simulink model "newfullgrid"  (R2024b)
settings: Solver=FixedStepDiscrete  StartTime=0.0  StopTime=24  FixedStep=0.0001  MaxStep=Ts  RelTol=1e-3
values from neighbouring files (symbols this model uses):
  C_boost = 1000e-6    (= 0.001)    [Full_system_design.m]    (also in systemdesigncode.m)
  f = 60    [Full_system_design.m]    (also in systemdesigncode.m)
  L_boost = 10*L_bound    (= 0.0016236346)    [Full_system_design.m]    (also in systemdesigncode.m)
  Lf = ((0.1*U^2)/(2*pi*f*(P/3)))    (= 0.00229819737825)    [Full_system_design.m]    (also in systemdesigncode.m)
  PV_power_max = Vpv_out_max * Ipv_out_max    (= 50729.7)    [Full_system_design.m]    (also in systemdesigncode.m)
  SOC_max = 90    [Full_system_design.m]    (also in batteryEnvLogic.m; gridrl.m = 1; systemdesigncode.m)
  SOC_min = 20    [Full_system_design.m]    (also in batteryEnvLogic.m; gridrl.m = 0.2; systemdesigncode.m)
  Solar_Irradiance = data.Solar_Irradiance    [systemdesigncode.m]
  Temperature = data.Temperature    [systemdesigncode.m]
  Ts = 10e-6    (= 1e-05)    [Full_system_design.m]    (also in systemdesigncode.m)
  V_bus_ref = 800    [Full_system_design.m]    (also in systemdesigncode.m)
undefined symbols (not defined in the file or in its folder): Active_Power_kW, Ion, Lithium
libraries: spsSeriesRLCBranchLib x6, slpidlib x4, spsMosfetLib x2, spsPWMGeneratorDCDCLib x2, rllib x2, spsPower3phInstantaneousLib x2, spsThreePhaseVIMeasurementLib x2, spsBatteryLib x1, spsCurrentMeasurementLib x1, spsDiodeLib x1, spsIGBTLib x1, spsPLL3phLib x1
settings Model: SimulationMode=accelerator  Creator=MohamedAbdallahMosta  LastModifiedBy=mac
settings DataIOCC: TimeSaveName=simTime  OutputSaveName=simOutput
settings DebuggingCC: UnconnectedInputMsg=warning  UnconnectedOutputMsg=warning  UnconnectedLineMsg=warning
settings ModelReferenceCC: EnableRefExpFcnMdlSchedulingChecks=on
settings RTWCC: GPUComputeCapability=3.5  DLArmComputeVersion=19.05

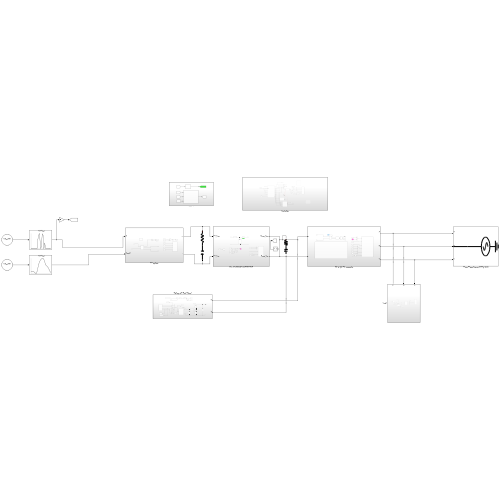
[thumbnail: Simulink's stored preview of the top-level diagram]
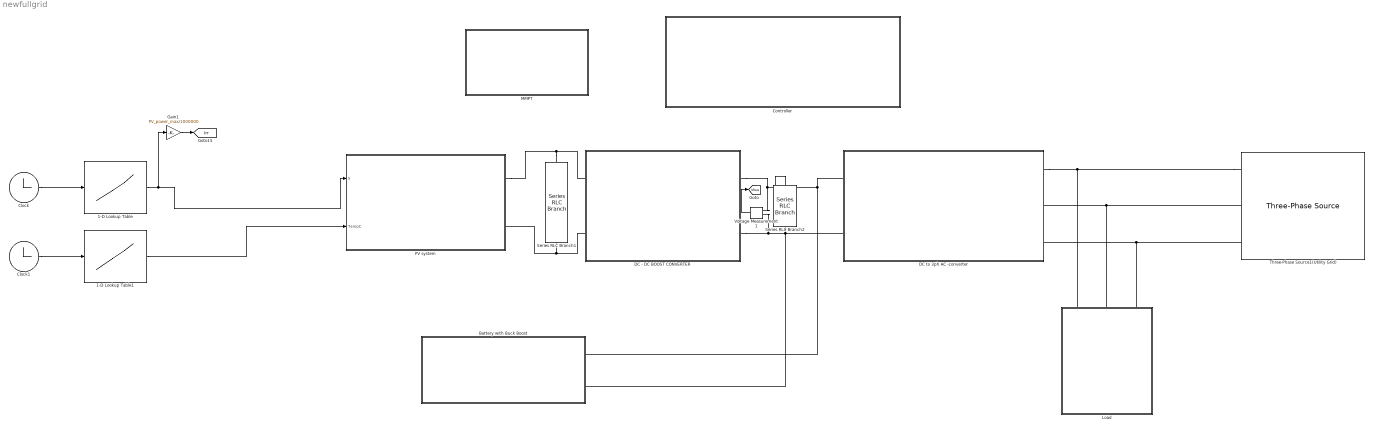
== system newfullgrid ==
  1-D Lookup Table : Lookup_n-D  NumberOfTableDimensions=1  BreakpointsForDimension1=[0:23]  Table=Solar_Irradiance  InternalRulePriority=Speed  RndMeth=Simplest
  1-D Lookup Table1 : Lookup_n-D  NumberOfTableDimensions=1  BreakpointsForDimension1=[0:23]  Table=Temperature  InternalRulePriority=Speed  RndMeth=Simplest
  Battery with Buck Boost : Subsystem
  Clock : Clock
  Clock1 : Clock
  Controller : Subsystem
  DC - DC BOOST CONVERTER : Subsystem
  DC to 3ph AC -converter : Subsystem
  Gain1 : Gain  Gain=PV_power_max/1000000
  Load : Subsystem
  MMPT : Subsystem
  PV system : Subsystem
  Series RLC Branch1 : spsSeriesRLCBranchLib/Series RLC Branch  LConnTagsString=__new0  RConnTagsString=__new0  BranchType=RC  Resistance=1e-4  Inductance=L_boost  SetiL0=off  InitialCurrent=0  Capacitance=100e-6  Setx0=off  InitialVoltage=406  Measurements=None
  Series RLC Branch2 : spsSeriesRLCBranchLib/Series RLC Branch  LConnTagsString=__new0  RConnTagsString=__new0  BranchType=RC  Resistance=1e-4  Inductance=L_boost  SetiL0=off  InitialCurrent=0  Capacitance=C_boost  Setx0=off  InitialVoltage=800  Measurements=None
  Three-Phase Source1(Utility Grid) : spsThreePhaseSourceLib/Three-Phase Source  InternalConnection=Yg  VoltagePhases=off  Voltage=380  PhaseAngle=0  Voltage_phases=[25e3 25e3 25e3]/sqrt(3)  PhaseAngles_phases=[0 -120 +120]  Frequency=f  NonIdealSource=off  SpecifyImpedance=off  Resistance=0.8929  Inductance=16.58e-3  ShortCircuitLevel=100e6  BaseVoltage=25e3  XRratio=7  BusType=swing  Pref=10e3  Qref=0  Prefabc=[10e3, 10e3, 10e3]  Qrefabc=[0, 0, 0]  Qmin=-inf  Qmax=inf
  Voltage Measurement1 : spsVoltageMeasurementLib/Voltage Measurement  PhasorSimulation=off  OutputType=Complex  PSBequivalent=0
  tag scope: Irr=global, Vbus=global
  wires:
  Gain1/1 -> [Irr]
  1-D Lookup Table1/1 -> PV system/2(TempC)
  Clock1/1 -> 1-D Lookup Table1/1
  Clock/1 -> 1-D Lookup Table/1
  1-D Lookup Table/1 -> PV system/1(S), Gain1/1
  Voltage Measurement1/1 -> [Vbus]
  connections:
  DC to 3ph AC -converter/RConn1 -- DC - DC BOOST CONVERTER/RConn1 -- Voltage Measurement1/LConn1 -- Series RLC Branch2/LConn1 -- Battery with Buck Boost/LConn1
  Series RLC Branch2/RConn1 -- Battery with Buck Boost/LConn2 -- DC to 3ph AC -converter/RConn2 -- DC - DC BOOST CONVERTER/RConn2 -- Voltage Measurement1/LConn2
  Series RLC Branch1/LConn1 -- DC - DC BOOST CONVERTER/LConn1 -- PV system/RConn1
  DC to 3ph AC -converter/LConn3 -- Three-Phase Source1(Utility Grid)/RConn3 -- Load/LConn3
  Three-Phase Source1(Utility Grid)/RConn1 -- DC to 3ph AC -converter/LConn1 -- Load/LConn1
  Three-Phase Source1(Utility Grid)/RConn2 -- Load/LConn2 -- DC to 3ph AC -converter/LConn2
  Series RLC Branch1/RConn1 -- DC - DC BOOST CONVERTER/LConn2 -- PV system/RConn2

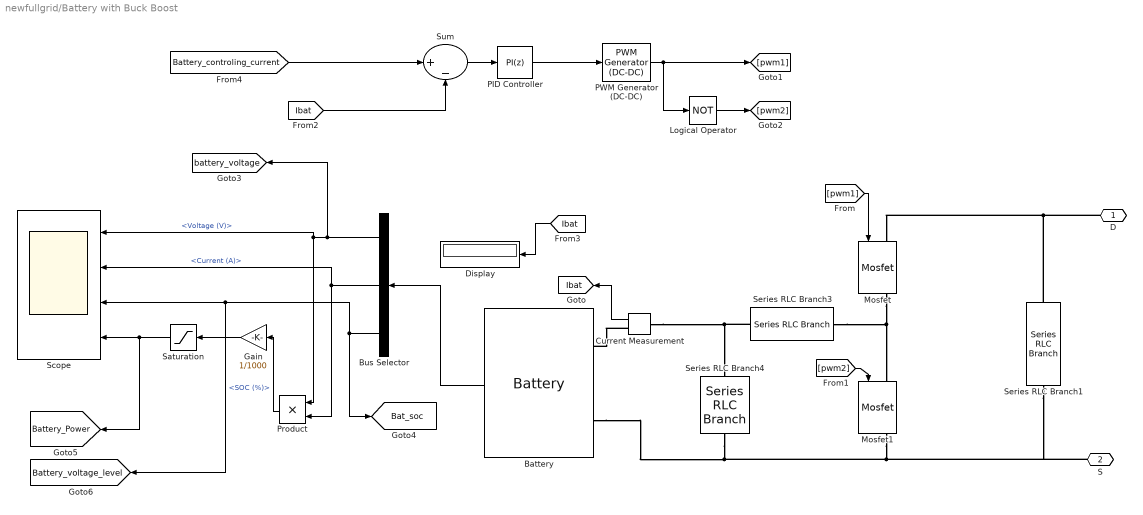
== system newfullgrid/Battery with Buck Boost ==
  Battery : spsBatteryLib/Battery  BatType=Lithium-Ion  NomV=360  NomQ=50  SOC=85  Batt_Tr=1  PresetModel=on  MaxQ=50  MinV=270  FullV=419.0354  Dis_rate=21.7391  R=0.072  Normal_OP=45.2174  expZone="[388.9389      2.456522]"
  Bus Selector : BusSelector  OutputSignals=Voltage (V),Current (A),SOC (%)
  Current Measurement : spsCurrentMeasurementLib/Current Measurement  PhasorSimulation=off  OutputType=Complex  PSBequivalent=0
  Display : Display
  Gain : Gain  Gain=1/1000
  Logical Operator : Logic  Operator=NOT  AllPortsSameDT=off  OutDataTypeStr=boolean
  Mosfet : spsMosfetLib/Mosfet  Ron=0.1  Lon=0  Rd=0.01  Vfd=0  IC=0  Rs=1e5  Cs=inf  Measurements=on
  Mosfet1 : spsMosfetLib/Mosfet  Ron=0.1  Lon=0  Rd=0.01  Vfd=0  IC=0  Rs=1e5  Cs=inf  Measurements=on
  PID Controller : slpidlib/PID Controller  Controller=PI  Form=Parallel  TimeDomain=Discrete-time  UseExternalTs=off  SampleTime=Ts  IntegratorMethod=Forward Euler  FilterMethod=Forward Euler  ControllerParametersSource=internal  P=1.5  I=25  UseKiTs=off  D=0  UseExternalDerivativeSource=off  N=100  UseFilter=on  TunerSelectOption=Transfer Function Based (PID Tuner App)  InitialConditionSource=internal  InitialConditionForIntegrator=0  InitialConditionForFilter=0  DifferentiatorICPrevScaledInput=0  ExternalReset=none  TrackingMode=off  Kt=1  LimitOutput=on  SatLimitsSource=internal  UpperSaturationLimit=0.95  LowerSaturationLimit=0  LinearizeAsGain=on  AntiWindupMode=none  Kb=1  LimitIntegrator=off  UpperIntegratorSaturationLimit=inf  LowerIntegratorSaturationLimit=-inf  POutMin=[]  POutMax=[]  IOutMin=[]  IOutMax=[]  DOutMin=[]  DOutMax=[]  NOutMin=[]  NOutMax=[]  SumOutMin=[]  SumOutMax=[]  SaturationOutMin=[]  SaturationOutMax=[]  PParamMin=[]  PParamMax=[]  IParamMin=[]  IParamMax=[]  DParamMin=[]  DParamMax=[]  NParamMin=[]  NParamMax=[]  KbParamMin=[]  KbParamMax=[]  KtParamMin=[]  KtParamMax=[]  KbOutMin=[]  KbOutMax=[]  KtOutMin=[]  KtOutMax=[]  IntegratorOutMin=[]  IntegratorOutMax=[]  FilterOutMin=[]  FilterOutMax=[]  SumI1OutMin=[]  SumI1OutMax=[]  SumI2OutMin=[]  SumI2OutMax=[]  SumI3OutMin=[]  SumI3OutMax=[]  SumI4OutMin=[]  SumI4OutMax=[]  SumDOutMin=[]  SumDOutMax=[]  DifferentiatorOutMin=[]  DifferentiatorOutMax=[]  FilterDiffOutCoefMin=[]  FilterDiffOutCoefMax=[]  ReciprocalOutMin=[]  ReciprocalOutMax=[]  SumDenOutMin=[]  SumDenOutMax=[]  SumNumOutMin=[]  SumNumOutMax=[]  DivideOutMin=[]  DivideOutMax=[]  UdiffTsProdOutMin=[]  UdiffTsProdOutMax=[]  NTsProdOutMin=[]  NTsProdOutMax=[]  UintegralTsProdOutMin=[]  UintegralTsProdOutMax=[]  UngainTsProdOutMin=[]  UngainTsProdOutMax=[]  ClampingZeroOutDataTypeStr=Inherit: Inherit via back propagation  ClampingZeroOutMin=[]  ClampingZeroOutMax=[]  FilterDenConstantOutDataTypeStr=Inherit: Inherit via back propagation  FilterDenConstantOutMin=[]  FilterDenConstantOutMax=[]  PCopyOutDataTypeStr=Inherit: Inherit via back propagation  PCopyOutMin=[]  PCopyOutMax=[]  NCopyOutDataTypeStr=Inherit: Inherit via back propagation  NCopyOutMin=[]  NCopyOutMax=[]  IntegratorContinuousStateAttributes=''  IntegratorStateMustResolveToSignalObject=off  IntegratorRTWStateStorageClass=Auto  FilterContinuousStateAttributes=''  FilterStateMustResolveToSignalObject=off  FilterRTWStateStorageClass=Auto  ParallelPVariant=InternalParameters  IdealPVariant=Disabled  IVariant=InternalParameters  DVariant=Disabled  IntegratorVariant=Discrete  SatVariant=Enabled  AWVariant=Passthrough  PCopyVariant=Disabled  TRVariant=Disabled  FdbkBlocksVariant=Forward  IdealPFdbkVariant=Disabled  SatFdbkVariant=Disabled  DerivativeFilterVariant=Disabled  NVariant=Disabled  NCopyVariant=Disabled_SignalSpec  FilterICVariant=Disabled  IntegratorICVariant=InternalICs  ExternalResetVariant=Disabled  TRSumVariant=Passthrough  SumFdbkVariant=Disabled  SumVariant=Sum_PI  TsampFilterVariant=InternalTs  TsampNgainVariant=Passthrough  TsampIntegralVariant=Disabled_SignalSpec  ExternalSaturationOutDataTypeStr=Inherit: Same as second input  DerivativeSourceVariant=Disabled  PreIntVariant=InternalPreInt
  PWM Generator (DC-DC) : spsPWMGeneratorDCDCLib/PWM Generator (DC-DC)  Fsw=5000  Ts=Ts
  Product : Product
  Saturation : Saturate  UpperLimit=30  LowerLimit=-30
  Scope : Scope  NumInputPorts=4
  Series RLC Branch1 : spsSeriesRLCBranchLib/Series RLC Branch  LConnTagsString=__new0  RConnTagsString=__new0  BranchType=RC  Resistance=1e-4  Inductance=13e-3  SetiL0=off  InitialCurrent=0  Capacitance=1000e-6  Setx0=off  InitialVoltage=0  Measurements=None
  Series RLC Branch3 : spsSeriesRLCBranchLib/Series RLC Branch  LConnTagsString=__new0  RConnTagsString=__new0  BranchType=RL  Resistance=1e-4  Inductance=13e-3  SetiL0=off  InitialCurrent=0  Capacitance=100e-6  Setx0=off  InitialVoltage=0  Measurements=None
  Series RLC Branch4 : spsSeriesRLCBranchLib/Series RLC Branch  LConnTagsString=__new0  RConnTagsString=__new0  BranchType=RC  Resistance=1e-4  Inductance=13e-3  SetiL0=off  InitialCurrent=0  Capacitance=20e-6  Setx0=off  InitialVoltage=0  Measurements=None
  Sum : Sum  Inputs=|+-
  D : PMIOPort  Side=Left
  S : PMIOPort  Port=2  Side=Left
  tag scope: Bat_soc=global, Battery_Power=global, Battery_voltage_level=global, Ibat=global, battery_voltage=global
  wires:
  [pwm1] -> Mosfet/1
  Bus Selector/1 -> [battery_voltage], Product/1, Scope/1  "<Voltage (V)>"
  [pwm2] -> Mosfet1/1
  Battery/1 -> Bus Selector/1
  Current Measurement/1 -> [Ibat]
  PID Controller/1 -> PWM Generator (DC-DC)/1
  Sum/1 -> PID Controller/1
  [Ibat] -> Sum/2
  PWM Generator (DC-DC)/1 -> Logical Operator/1, [pwm1]
  [Ibat] -> Display/1
  Logical Operator/1 -> [pwm2]
  Bus Selector/2 -> Product/2, Scope/2  "<Current (A)>"
  Bus Selector/3 -> [Bat_soc], [Battery_voltage_level], Scope/3  "<SOC (%)>"
  Product/1 -> Gain/1
  [Battery_controling_current] -> Sum/1
  Gain/1 -> Saturation/1
  Saturation/1 -> [Battery_Power], Scope/4
  connections:
  Series RLC Branch3/RConn1 -- Current Measurement/LConn1 -- Series RLC Branch4/LConn1
  Series RLC Branch4/RConn1 -- Battery/LConn2 -- Series RLC Branch1/RConn1 -- S/RConn1 -- Mosfet1/RConn1
  Mosfet/RConn1 -- Series RLC Branch3/LConn1 -- Mosfet1/LConn1
  Current Measurement/RConn1 -- Battery/LConn1
  D/RConn1 -- Series RLC Branch1/LConn1 -- Mosfet/LConn1

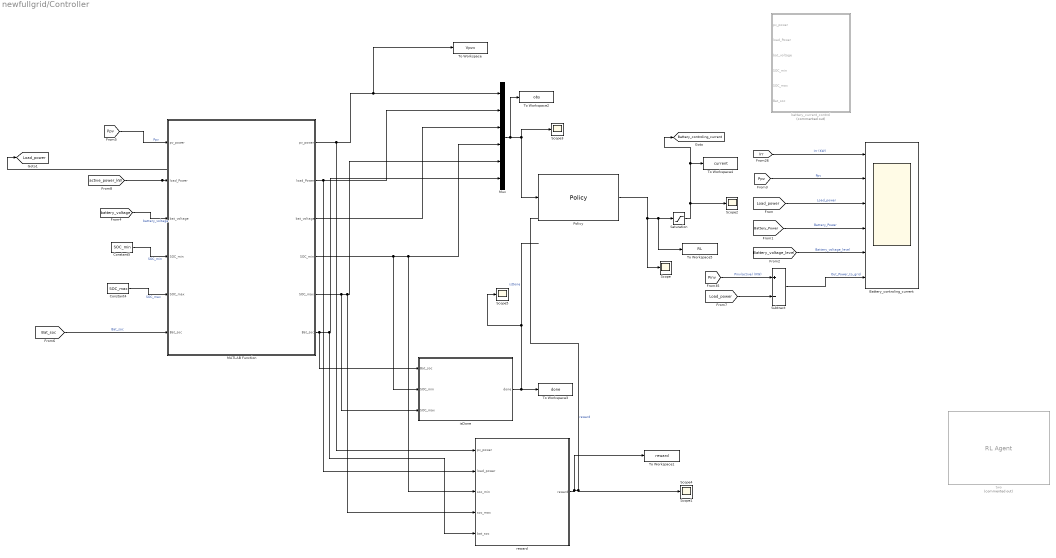
== system newfullgrid/Controller ==
  Battery_controling_current : Scope  NumInputPorts=6
  Constant4 : Constant  Value=SOC_max
  Constant5 : Constant  Value=SOC_min
  MATLAB Function : MATLAB Function  TreatAsAtomicUnit=on
  Mux : Mux  Inputs=6
  Policy : rllib/Policy  MATFile=policyData.mat  PolicyParamsAsInput=off  PolicyParamsBusName=policy_param_bus  SimUsingCodegen=off
  Saturation : Saturate  UpperLimit=+86.95  LowerLimit=-86.95
  Scope{,1..5} (6 alike) : Scope
  Subtract : Sum  Inputs=+-
  To Workspace : ToWorkspace  VariableName=Vpvv  SampleTime=-1
  To Workspace1 : ToWorkspace  VariableName=reward  SampleTime=-1
  To Workspace2 : ToWorkspace  VariableName=obs  SampleTime=-1
  To Workspace3 : ToWorkspace  VariableName=done  SampleTime=-1
  To Workspace4 : ToWorkspace  VariableName=current  SampleTime=-1
  To Workspace5 : ToWorkspace  VariableName=RL  SampleTime=-1
  battery_current_control : MATLAB Function  Commented=on  TreatAsAtomicUnit=on
  isDone : MATLAB Function  TreatAsAtomicUnit=on
  "reward " : MATLAB Function  TreatAsAtomicUnit=on
  two : rllib/RL Agent  Commented=on  Agent=agent  ExternalActionAsInput=off  ProvideLastAction=off  ProvideCumRwd=off  TreatAsDirectFeedthrough=on  UseStrictObservationDataTypes=off
  tag scope: Battery_controling_current=global, Load_power=global
  wires:
  Saturation/1 -> [Battery_controling_current], To Workspace4/1, Scope2/1
  [Pinv] -> Subtract/1  "Pinv(active) (KW)"
  [Load_power] -> Subtract/2
  [Irr] -> Battery_controling_current/1  "Irr (KW)"
  [Ppv] -> Battery_controling_current/2  "Ppv"
  [Load_power] -> Battery_controling_current/3  "Load_power"
  [Battery_Power] -> Battery_controling_current/4  "Battery_Power"
  [Battery_voltage_level] -> Battery_controling_current/5  "Battery_voltage_level"
  Subtract/1 -> Battery_controling_current/6  "Out_Power_to_grid"
  isDone/1(done) -> Scope5/1, To Workspace3/1  "isDone"
  "reward "/1(reward) -> To Workspace1/1, Scope1/1  "reward"
  [Ppv] -> MATLAB Function/1("pv_power ")  "Ppv"
  [active_power_kW] -> [Load_power], MATLAB Function/2("load_Power ")
  [battery_voltage] -> MATLAB Function/3("bat_voltage ")  "battery_voltage"
  Constant5/1 -> MATLAB Function/4("SOC_min ")  "SOC_min"
  Constant4/1 -> MATLAB Function/5("SOC_max ")  "SOC_max"
  [Bat_soc] -> MATLAB Function/6("Bat_soc ")  "Bat_soc"
  Policy/1 -> Scope/1, To Workspace5/1, Saturation/1
  Mux/1 -> To Workspace2/1, Policy/1, Scope3/1
  MATLAB Function/1(pv_power) -> "reward "/1(pv_power), To Workspace/1, Mux/1
  MATLAB Function/2(load_Power) -> "reward "/2(load_power), Mux/2
  MATLAB Function/3(bat_voltage) -> Mux/3
  MATLAB Function/4(SOC_min) -> isDone/2(SOC_min), "reward "/3(soc_min), Mux/4
  MATLAB Function/5(SOC_max) -> isDone/3(SOC_max), "reward "/4(soc_max), Mux/5
  MATLAB Function/6(Bat_soc) -> isDone/1(Bat_soc), "reward "/5(bat_soc), Mux/6

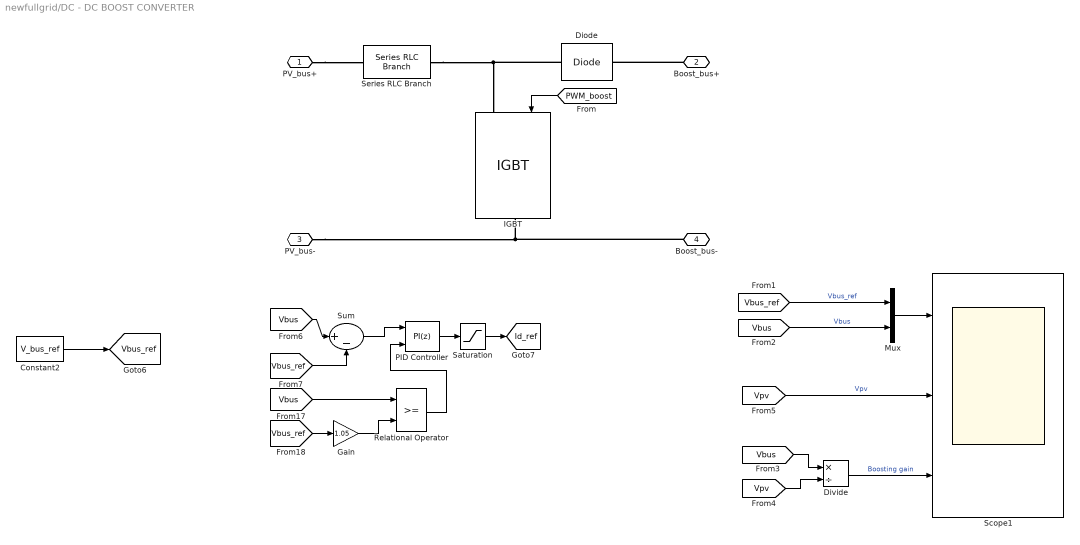
== system newfullgrid/DC - DC BOOST CONVERTER ==
  Constant2 : Constant  Value=V_bus_ref
  Diode : spsDiodeLib/Diode  Ron=0.001  Lon=0  Vf=0.8  IC=0  UseSnubber=0  Rs=500  Cs=250e-9  Measurements=off
  Divide : Product  Inputs=*/
  Gain : Gain  Gain=1.05
  IGBT : spsIGBTLib/IGBT  Ron=0.001  Lon=0  Vf=1  Tf=1e-6  Tt=2e-6  IC=0  Rs=1e5  Cs=inf  Measurements=off
  Mux : Mux  Inputs=2
  PID Controller : slpidlib/PID Controller  Controller=PI  Form=Parallel  TimeDomain=Discrete-time  UseExternalTs=off  SampleTime=20*Ts  IntegratorMethod=Forward Euler  FilterMethod=Forward Euler  ControllerParametersSource=internal  P=0.15  I=80  UseKiTs=off  D=0  UseExternalDerivativeSource=off  N=100  UseFilter=on  TunerSelectOption=Transfer Function Based (PID Tuner App)  InitialConditionSource=internal  InitialConditionForIntegrator=0  InitialConditionForFilter=0  DifferentiatorICPrevScaledInput=0  ExternalReset=rising  TrackingMode=off  Kt=1  LimitOutput=off  SatLimitsSource=internal  UpperSaturationLimit=inf  LowerSaturationLimit=-inf  LinearizeAsGain=on  AntiWindupMode=none  Kb=1  LimitIntegrator=off  UpperIntegratorSaturationLimit=inf  LowerIntegratorSaturationLimit=-inf  POutMin=[]  POutMax=[]  IOutMin=[]  IOutMax=[]  DOutMin=[]  DOutMax=[]  NOutMin=[]  NOutMax=[]  SumOutMin=[]  SumOutMax=[]  SaturationOutMin=[]  SaturationOutMax=[]  PParamMin=[]  PParamMax=[]  IParamMin=[]  IParamMax=[]  DParamMin=[]  DParamMax=[]  NParamMin=[]  NParamMax=[]  KbParamMin=[]  KbParamMax=[]  KtParamMin=[]  KtParamMax=[]  KbOutMin=[]  KbOutMax=[]  KtOutMin=[]  KtOutMax=[]  IntegratorOutMin=[]  IntegratorOutMax=[]  FilterOutMin=[]  FilterOutMax=[]  SumI1OutMin=[]  SumI1OutMax=[]  SumI2OutMin=[]  SumI2OutMax=[]  SumI3OutMin=[]  SumI3OutMax=[]  SumI4OutMin=[]  SumI4OutMax=[]  SumDOutMin=[]  SumDOutMax=[]  DifferentiatorOutMin=[]  DifferentiatorOutMax=[]  FilterDiffOutCoefMin=[]  FilterDiffOutCoefMax=[]  ReciprocalOutMin=[]  ReciprocalOutMax=[]  SumDenOutMin=[]  SumDenOutMax=[]  SumNumOutMin=[]  SumNumOutMax=[]  DivideOutMin=[]  DivideOutMax=[]  UdiffTsProdOutMin=[]  UdiffTsProdOutMax=[]  NTsProdOutMin=[]  NTsProdOutMax=[]  UintegralTsProdOutMin=[]  UintegralTsProdOutMax=[]  UngainTsProdOutMin=[]  UngainTsProdOutMax=[]  ClampingZeroOutDataTypeStr=Inherit: Inherit via back propagation  ClampingZeroOutMin=[]  ClampingZeroOutMax=[]  FilterDenConstantOutDataTypeStr=Inherit: Inherit via back propagation  FilterDenConstantOutMin=[]  FilterDenConstantOutMax=[]  PCopyOutDataTypeStr=Inherit: Inherit via back propagation  PCopyOutMin=[]  PCopyOutMax=[]  NCopyOutDataTypeStr=Inherit: Inherit via back propagation  NCopyOutMin=[]  NCopyOutMax=[]  IntegratorContinuousStateAttributes=''  IntegratorStateMustResolveToSignalObject=off  IntegratorRTWStateStorageClass=Auto  FilterContinuousStateAttributes=''  FilterStateMustResolveToSignalObject=off  FilterRTWStateStorageClass=Auto  ParallelPVariant=InternalParameters  IdealPVariant=Disabled  IVariant=InternalParameters  DVariant=Disabled  IntegratorVariant=Discrete  SatVariant=Disabled  AWVariant=Passthrough  PCopyVariant=Disabled  TRVariant=Disabled  FdbkBlocksVariant=Forward  IdealPFdbkVariant=Disabled  SatFdbkVariant=Disabled  DerivativeFilterVariant=Disabled  NVariant=Disabled  NCopyVariant=Disabled_SignalSpec  FilterICVariant=Disabled  IntegratorICVariant=InternalICs  ExternalResetVariant=ExternalReset  TRSumVariant=Passthrough  SumFdbkVariant=Disabled  SumVariant=Sum_PI  TsampFilterVariant=InternalTs  TsampNgainVariant=Passthrough  TsampIntegralVariant=Disabled_SignalSpec  ExternalSaturationOutDataTypeStr=Inherit: Same as second input  DerivativeSourceVariant=Disabled  PreIntVariant=InternalPreInt
  Relational Operator : RelationalOperator  OutDataTypeStr=boolean  RndMeth=Simplest  InputSameDT=off
  Saturation : Saturate  UpperLimit=150  LowerLimit=-150
  Scope1 : Scope  NumInputPorts=3
  Series RLC Branch : spsSeriesRLCBranchLib/Series RLC Branch  LConnTagsString=__new0  RConnTagsString=__new0  BranchType=L  Resistance=1  Inductance=L_boost  SetiL0=off  InitialCurrent=0  Capacitance=1e-6  Setx0=off  InitialVoltage=0  Measurements=None
  Sum : Sum  Inputs=|+-
  PV_bus+ : PMIOPort  Side=Left
  Boost_bus+ : PMIOPort  Port=2  Side=Right
  PV_bus- : PMIOPort  Port=3  Side=Left
  Boost_bus- : PMIOPort  Port=4  Side=Right
  tag scope: Id_ref=global, Vbus_ref=global
  wires:
  [PWM_boost] -> IGBT/1
  [Vbus] -> Divide/1
  [Vpv] -> Divide/2
  Divide/1 -> Scope1/3  "Boosting gain"
  Constant2/1 -> [Vbus_ref]
  [Vbus] -> Relational Operator/1
  PID Controller/1 -> Saturation/1
  [Vbus_ref] -> Gain/1
  Sum/1 -> PID Controller/1
  [Vbus] -> Sum/1
  [Vbus_ref] -> Sum/2
  Saturation/1 -> [Id_ref]
  Relational Operator/1 -> PID Controller/2
  Gain/1 -> Relational Operator/2
  [Vbus_ref] -> Mux/1  "Vbus_ref"
  [Vbus] -> Mux/2  "Vbus"
  Mux/1 -> Scope1/1
  [Vpv] -> Scope1/2  "Vpv"
  connections:
  Series RLC Branch/RConn1 -- Diode/LConn1 -- IGBT/LConn1
  PV_bus-/RConn1 -- Boost_bus-/RConn1 -- IGBT/RConn1
  PV_bus+/RConn1 -- Series RLC Branch/LConn1
  Boost_bus+/RConn1 -- Diode/RConn1

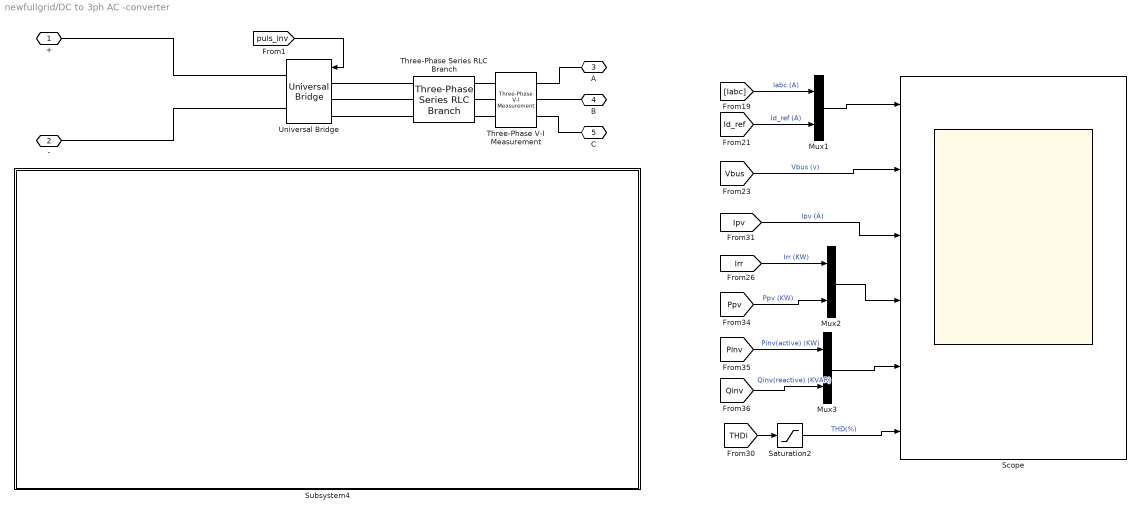
== system newfullgrid/DC to 3ph AC -converter ==
  Mux1 : Mux  Inputs=2
  Mux2 : Mux  Inputs=2
  Mux3 : Mux  Inputs=2
  Saturation2 : Saturate  UpperLimit=15  LowerLimit=0
  Scope : Scope  NumInputPorts=6
  Subsystem4 : Subsystem
  Three-Phase Series RLC Branch : spsThreePhaseSeriesRLCBranchLib/Three-Phase Series RLC Branch  LConnTagsString=A|B|C  RConnTagsString=A|B|C  BranchType=L  Resistance=1  Inductance=Lf  Capacitance=1e-6  Measurements=None
  Three-Phase V-I Measurement : spsThreePhaseVIMeasurementLib/Three-Phase V-I Measurement  VoltageMeasurement=phase-to-ground  SetLabelV=on  LabelV=Vabc  Vpu=off  VpuLL=off  CurrentMeasurement=yes  SetLabelI=on  LabelI=Iabc  Ipu=off  Pbase=100e6  Vbase=500e3  OutputType=Complex  PhasorSimulation=off  PSBequivalent=0
  Universal Bridge : spsUniversalBridgeLib/Universal Bridge  Arms=3  SnubberResistance=1e5  SnubberCapacitance=inf  Device=IGBT / Diodes  Ron=1e-3  Lon=0  ForwardVoltages="[  0  0  ]"  ForwardVoltage=0  GTOparameters=[ 10e-6 , 20e-6 ]  IGBTparameters=[ 1e-6 , 2e-6 ]  Measurements=None  Measurements_2=None  converterType=Rectifier
  + : PMIOPort  Side=Right
  - : PMIOPort  Port=2  Side=Right
  A : PMIOPort  Port=3  Side=Left
  B : PMIOPort  Port=4  Side=Left
  C : PMIOPort  Port=5  Side=Left
  wires:
  [puls_inv] -> Universal Bridge/1
  [Ppv] -> Mux2/2  "Ppv (KW)"
  [Iabc] -> Mux1/1  "Iabc (A)"
  [Qinv] -> Mux3/2  "Qinv(reactive) (KVAR)"
  Saturation2/1 -> Scope/6  "THD(%)"
  [Pinv] -> Mux3/1  "Pinv(active) (KW)"
  [Vbus] -> Scope/2  "Vbus (v)"
  [THDi] -> Saturation2/1
  Mux1/1 -> Scope/1
  Mux3/1 -> Scope/5
  [Irr] -> Mux2/1  "Irr (KW)"
  [Id_ref] -> Mux1/2  "Id_ref (A)"
  [Ipv] -> Scope/3  "Ipv (A)"
  Mux2/1 -> Scope/4
  connections:
  Universal Bridge/RConn1 -- +/RConn1
  Three-Phase Series RLC Branch/RConn2 -- Three-Phase V-I Measurement/LConn2
  Three-Phase Series RLC Branch/RConn3 -- Three-Phase V-I Measurement/LConn3
  Universal Bridge/LConn1 -- Three-Phase Series RLC Branch/LConn1
  Universal Bridge/LConn2 -- Three-Phase Series RLC Branch/LConn2
  Universal Bridge/LConn3 -- Three-Phase Series RLC Branch/LConn3
  Three-Phase V-I Measurement/LConn1 -- Three-Phase Series RLC Branch/RConn1
  Universal Bridge/RConn2 -- -/RConn1
  A/RConn1 -- Three-Phase V-I Measurement/RConn1
  Three-Phase V-I Measurement/RConn2 -- B/RConn1
  Three-Phase V-I Measurement/RConn3 -- C/RConn1

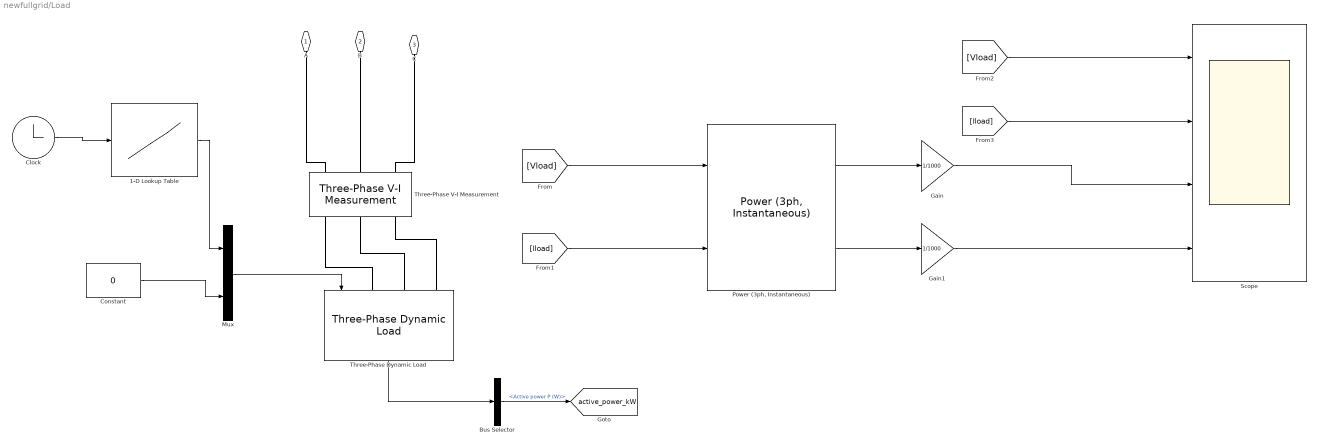
== system newfullgrid/Load ==
  1-D Lookup Table : Lookup_n-D  NumberOfTableDimensions=1  BreakpointsForDimension1=[0:23]  Table=Active_Power_kW  InternalRulePriority=Speed  RndMeth=Simplest
  Bus Selector : BusSelector  OutputSignals=Active power P (W)
  Clock : Clock
  Constant : Constant  Value=0
  Gain : Gain  Gain=1/1000
  Gain1 : Gain  Gain=1/1000
  Mux : Mux  Inputs=2
  "Power (3ph, Instantaneous)" : spsPower3phInstantaneousLib/Power (3ph, Instantaneous)
  Scope : Scope  NumInputPorts=4
  Three-Phase Dynamic Load : spsThreePhaseDynamicLoadLib/Three-Phase Dynamic Load  NominalVoltage=[ 380 60 ]  ActiveReactivePowers=[10e6 0]  PositiveSequence=[0.994 -11.8]  ExternalControl=on  NpNq=[1.3 2]  TimeConstants="[0  0  0  0]"  MinimumVoltage=0.7  Tfilter=1e-4  LoadFlowParameters=[4,0,0,0,0]
  Three-Phase V-I Measurement : spsThreePhaseVIMeasurementLib/Three-Phase V-I Measurement  VoltageMeasurement=phase-to-ground  SetLabelV=on  LabelV=Vload  Vpu=off  VpuLL=off  CurrentMeasurement=yes  SetLabelI=on  LabelI=Iload  Ipu=off  Pbase=100e6  Vbase=500e3  OutputType=Complex  PhasorSimulation=off  PSBequivalent=0
  A : PMIOPort  Side=Left
  B : PMIOPort  Port=2  Side=Left
  C : PMIOPort  Port=3  Side=Left
  tag scope: active_power_kW=global
  wires:
  [Vload] -> "Power (3ph, Instantaneous)"/1
  [Iload] -> "Power (3ph, Instantaneous)"/2
  "Power (3ph, Instantaneous)"/1 -> Gain/1
  "Power (3ph, Instantaneous)"/2 -> Gain1/1
  [Vload] -> Scope/1
  [Iload] -> Scope/2
  Gain/1 -> Scope/3
  Gain1/1 -> Scope/4
  Three-Phase Dynamic Load/1 -> Bus Selector/1
  Clock/1 -> 1-D Lookup Table/1
  Constant/1 -> Mux/2
  1-D Lookup Table/1 -> Mux/1
  Mux/1 -> Three-Phase Dynamic Load/1
  Bus Selector/1 -> [active_power_kW]  "<Active power P (W)>"
  connections:
  Three-Phase V-I Measurement/LConn3 -- C/RConn1
  Three-Phase V-I Measurement/RConn1 -- Three-Phase Dynamic Load/LConn1
  Three-Phase V-I Measurement/LConn1 -- A/RConn1
  Three-Phase V-I Measurement/RConn2 -- Three-Phase Dynamic Load/LConn2
  Three-Phase V-I Measurement/LConn2 -- B/RConn1
  Three-Phase V-I Measurement/RConn3 -- Three-Phase Dynamic Load/LConn3

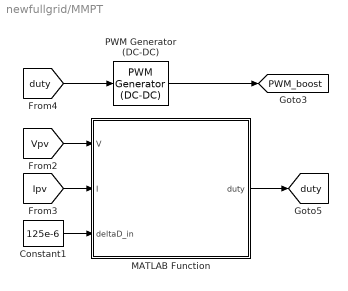
== system newfullgrid/MMPT ==
  Constant1 : Constant  Value=125e-6
  MATLAB Function : MATLAB Function  TreatAsAtomicUnit=on
  PWM Generator (DC-DC) : spsPWMGeneratorDCDCLib/PWM Generator (DC-DC)  Fsw=5000  Ts=Ts
  tag scope: PWM_boost=global, duty=global
  wires:
  PWM Generator (DC-DC)/1 -> [PWM_boost]
  Constant1/1 -> MATLAB Function/3(deltaD_in)
  [Vpv] -> MATLAB Function/1(V)
  [Ipv] -> MATLAB Function/2(I)
  MATLAB Function/1(duty) -> [duty]
  [duty] -> PWM Generator (DC-DC)/1

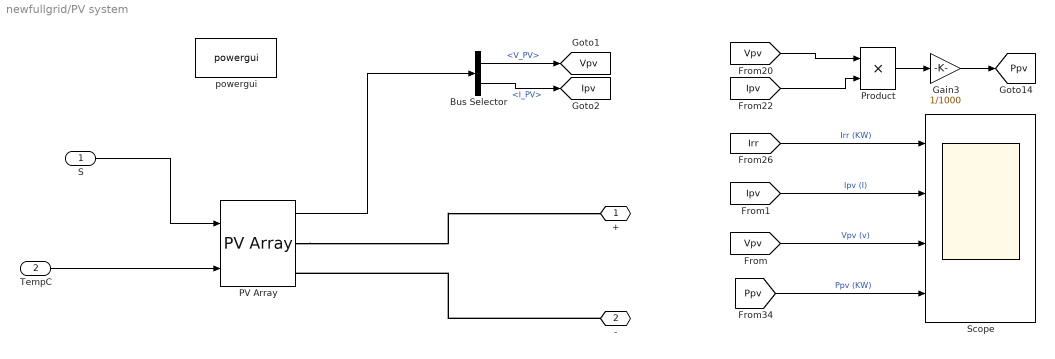
== system newfullgrid/PV system ==
  S : Inport
  TempC : Inport  Port=2
  Bus Selector : BusSelector  OutputSignals=V_PV,I_PV
  Gain3 : Gain  Gain=1/1000
  PV Array : spsPVArrayLib/PV Array  Npar=no_parrell_PV_units  Nser=no_series_PV_units  PlotType=array @ 1000 W/m2 & specified temperatures  S_vec="[ 1000  500  100 ]"  Temp_C_vec="[ 45 25  ]"  ModuleName=User-defined  PlotWhenSelected=off  Pm=213.15  Ncell=60  Voc=36.3  Isc=7.84  Vm=29  Im=7.35  beta_Voc_pc=-0.36099  alpha_Isc_pc=0.102  beta_Voc=-0.13104  alpha_Isc=0.0079968  IL=7.8654  I0=2.9273e-10  nI=0.98119  Rsh=313.0553  Rs=0.39381  RobustModel=off  RobustCellTemperature=313.3991  BAL=on  Tc=1e-6  Tfilter=5e-5
  Product : Product
  Scope : Scope  NumInputPorts=4
  powergui : spspowerguiLib/powergui  Priority=1  SimulationMode=Discrete  SampleTime=Ts  frequency=60  Iterations=50  frequencyindice=0  Pbase=100e6  ErrMax=1e-4  UnitsV=kV  UnitsW=MW  buscounter=0  FunctionMessages=off  echomessages=off  EnableUseOfTLC=off  CurrentSourceSwitches=off  DisableSnubberDevices=off  DisableRonSwitches=off  DisableVfSwitches=off  DisplayEquations=off  AutomaticDiscreteSolvers=off  SolverType=Tustin/Backward Euler (TBE)  Interpol=off  ExternalGateDelay=off  methode=off  Ts=100  x0status=blocks  SPID=on  SwTol=0  HookPort=off  NonlinearTolerance=1e-4  nMaxIteration=100  ContinueOnMaxIteration=off  RestoreLinks=warning  ResistiveCurrentMeasurement=off  Frange=[0:2:500]  Ylog=off  Xlog=on  ShowGrid=off  save=off  variable=ZData  structure=0  ZoomFFT=off  StartTime=0.0  cycles=1  DisplayStyle=1  fundamental=60  FreqAxis=off  MaxFrequency=1000  frequencyindicesteady=1  RmsSteady=1  display=off
  + : PMIOPort  Side=Right
  - : PMIOPort  Port=2  Side=Right
  tag scope: Ipv=global, Ppv=global, Vpv=global
  wires:
  [Irr] -> Scope/1  "Irr (KW)"
  [Vpv] -> Product/1
  [Vpv] -> Scope/3  "Vpv (v)"
  [Ipv] -> Product/2
  Product/1 -> Gain3/1
  [Ppv] -> Scope/4  "Ppv (KW)"
  Gain3/1 -> [Ppv]
  [Ipv] -> Scope/2  "Ipv (I)"
  Bus Selector/1 -> [Vpv]  "<V_PV>"
  Bus Selector/2 -> [Ipv]  "<I_PV>"
  PV Array/1 -> Bus Selector/1
  TempC/1 -> PV Array/2
  S/1 -> PV Array/1
  connections:
  PV Array/RConn1 -- +/RConn1
  -/RConn1 -- PV Array/RConn2

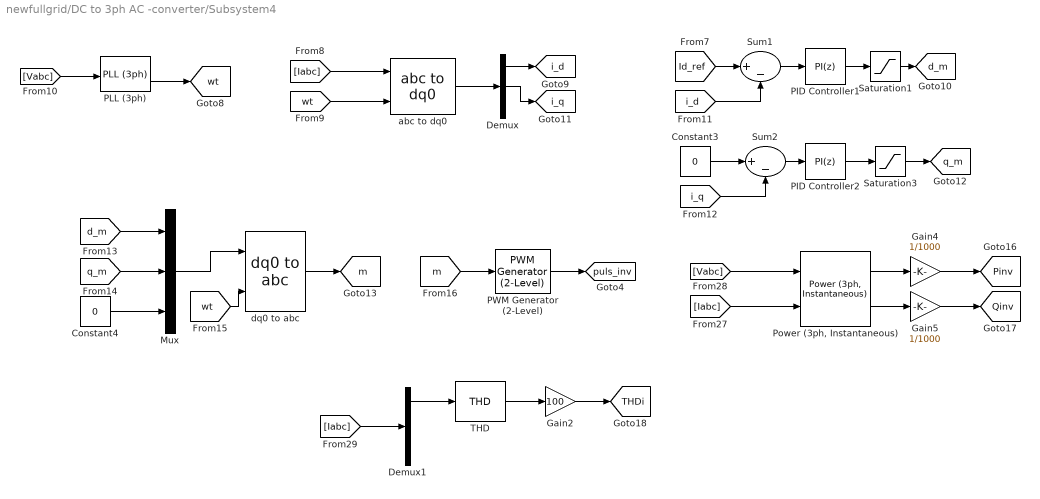
== system newfullgrid/DC to 3ph AC -converter/Subsystem4 ==
  Constant3 : Constant  Value=0
  Constant4 : Constant  Value=0
  Demux : Demux  Outputs=3
  Demux1 : Demux  Outputs=3
  Gain2 : Gain  Gain=100
  Gain4 : Gain  Gain=1/1000
  Gain5 : Gain  Gain=1/1000
  Mux : Mux  Inputs=3
  PID Controller1 : slpidlib/PID Controller  Controller=PI  Form=Parallel  TimeDomain=Discrete-time  UseExternalTs=off  SampleTime=Ts  IntegratorMethod=Forward Euler  FilterMethod=Forward Euler  ControllerParametersSource=internal  P=0.005  I=1  UseKiTs=off  D=0  UseExternalDerivativeSource=off  N=100  UseFilter=on  TunerSelectOption=Transfer Function Based (PID Tuner App)  InitialConditionSource=internal  InitialConditionForIntegrator=0  InitialConditionForFilter=0  DifferentiatorICPrevScaledInput=0  ExternalReset=none  TrackingMode=off  Kt=1  LimitOutput=off  SatLimitsSource=internal  UpperSaturationLimit=inf  LowerSaturationLimit=-inf  LinearizeAsGain=on  AntiWindupMode=none  Kb=1  LimitIntegrator=off  UpperIntegratorSaturationLimit=inf  LowerIntegratorSaturationLimit=-inf  POutMin=[]  POutMax=[]  IOutMin=[]  IOutMax=[]  DOutMin=[]  DOutMax=[]  NOutMin=[]  NOutMax=[]  SumOutMin=[]  SumOutMax=[]  SaturationOutMin=[]  SaturationOutMax=[]  PParamMin=[]  PParamMax=[]  IParamMin=[]  IParamMax=[]  DParamMin=[]  DParamMax=[]  NParamMin=[]  NParamMax=[]  KbParamMin=[]  KbParamMax=[]  KtParamMin=[]  KtParamMax=[]  KbOutMin=[]  KbOutMax=[]  KtOutMin=[]  KtOutMax=[]  IntegratorOutMin=[]  IntegratorOutMax=[]  FilterOutMin=[]  FilterOutMax=[]  SumI1OutMin=[]  SumI1OutMax=[]  SumI2OutMin=[]  SumI2OutMax=[]  SumI3OutMin=[]  SumI3OutMax=[]  SumI4OutMin=[]  SumI4OutMax=[]  SumDOutMin=[]  SumDOutMax=[]  DifferentiatorOutMin=[]  DifferentiatorOutMax=[]  FilterDiffOutCoefMin=[]  FilterDiffOutCoefMax=[]  ReciprocalOutMin=[]  ReciprocalOutMax=[]  SumDenOutMin=[]  SumDenOutMax=[]  SumNumOutMin=[]  SumNumOutMax=[]  DivideOutMin=[]  DivideOutMax=[]  UdiffTsProdOutMin=[]  UdiffTsProdOutMax=[]  NTsProdOutMin=[]  NTsProdOutMax=[]  UintegralTsProdOutMin=[]  UintegralTsProdOutMax=[]  UngainTsProdOutMin=[]  UngainTsProdOutMax=[]  ClampingZeroOutDataTypeStr=Inherit: Inherit via back propagation  ClampingZeroOutMin=[]  ClampingZeroOutMax=[]  FilterDenConstantOutDataTypeStr=Inherit: Inherit via back propagation  FilterDenConstantOutMin=[]  FilterDenConstantOutMax=[]  PCopyOutDataTypeStr=Inherit: Inherit via back propagation  PCopyOutMin=[]  PCopyOutMax=[]  NCopyOutDataTypeStr=Inherit: Inherit via back propagation  NCopyOutMin=[]  NCopyOutMax=[]  IntegratorContinuousStateAttributes=''  IntegratorStateMustResolveToSignalObject=off  IntegratorRTWStateStorageClass=Auto  FilterContinuousStateAttributes=''  FilterStateMustResolveToSignalObject=off  FilterRTWStateStorageClass=Auto  ParallelPVariant=InternalParameters  IdealPVariant=Disabled  IVariant=InternalParameters  DVariant=Disabled  IntegratorVariant=Discrete  SatVariant=Disabled  AWVariant=Passthrough  PCopyVariant=Disabled  TRVariant=Disabled  FdbkBlocksVariant=Forward  IdealPFdbkVariant=Disabled  SatFdbkVariant=Disabled  DerivativeFilterVariant=Disabled  NVariant=Disabled  NCopyVariant=Disabled_SignalSpec  FilterICVariant=Disabled  IntegratorICVariant=InternalICs  ExternalResetVariant=Disabled  TRSumVariant=Passthrough  SumFdbkVariant=Disabled  SumVariant=Sum_PI  TsampFilterVariant=InternalTs  TsampNgainVariant=Passthrough  TsampIntegralVariant=Disabled_SignalSpec  ExternalSaturationOutDataTypeStr=Inherit: Same as second input  DerivativeSourceVariant=Disabled  PreIntVariant=InternalPreInt
  PID Controller2 : slpidlib/PID Controller  Controller=PI  Form=Parallel  TimeDomain=Discrete-time  UseExternalTs=off  SampleTime=Ts  IntegratorMethod=Forward Euler  FilterMethod=Forward Euler  ControllerParametersSource=internal  P=0.01  I=1  UseKiTs=off  D=0  UseExternalDerivativeSource=off  N=100  UseFilter=on  TunerSelectOption=Transfer Function Based (PID Tuner App)  InitialConditionSource=internal  InitialConditionForIntegrator=0  InitialConditionForFilter=0  DifferentiatorICPrevScaledInput=0  ExternalReset=none  TrackingMode=off  Kt=1  LimitOutput=off  SatLimitsSource=internal  UpperSaturationLimit=inf  LowerSaturationLimit=-inf  LinearizeAsGain=on  AntiWindupMode=none  Kb=1  LimitIntegrator=off  UpperIntegratorSaturationLimit=inf  LowerIntegratorSaturationLimit=-inf  POutMin=[]  POutMax=[]  IOutMin=[]  IOutMax=[]  DOutMin=[]  DOutMax=[]  NOutMin=[]  NOutMax=[]  SumOutMin=[]  SumOutMax=[]  SaturationOutMin=[]  SaturationOutMax=[]  PParamMin=[]  PParamMax=[]  IParamMin=[]  IParamMax=[]  DParamMin=[]  DParamMax=[]  NParamMin=[]  NParamMax=[]  KbParamMin=[]  KbParamMax=[]  KtParamMin=[]  KtParamMax=[]  KbOutMin=[]  KbOutMax=[]  KtOutMin=[]  KtOutMax=[]  IntegratorOutMin=[]  IntegratorOutMax=[]  FilterOutMin=[]  FilterOutMax=[]  SumI1OutMin=[]  SumI1OutMax=[]  SumI2OutMin=[]  SumI2OutMax=[]  SumI3OutMin=[]  SumI3OutMax=[]  SumI4OutMin=[]  SumI4OutMax=[]  SumDOutMin=[]  SumDOutMax=[]  DifferentiatorOutMin=[]  DifferentiatorOutMax=[]  FilterDiffOutCoefMin=[]  FilterDiffOutCoefMax=[]  ReciprocalOutMin=[]  ReciprocalOutMax=[]  SumDenOutMin=[]  SumDenOutMax=[]  SumNumOutMin=[]  SumNumOutMax=[]  DivideOutMin=[]  DivideOutMax=[]  UdiffTsProdOutMin=[]  UdiffTsProdOutMax=[]  NTsProdOutMin=[]  NTsProdOutMax=[]  UintegralTsProdOutMin=[]  UintegralTsProdOutMax=[]  UngainTsProdOutMin=[]  UngainTsProdOutMax=[]  ClampingZeroOutDataTypeStr=Inherit: Inherit via back propagation  ClampingZeroOutMin=[]  ClampingZeroOutMax=[]  FilterDenConstantOutDataTypeStr=Inherit: Inherit via back propagation  FilterDenConstantOutMin=[]  FilterDenConstantOutMax=[]  PCopyOutDataTypeStr=Inherit: Inherit via back propagation  PCopyOutMin=[]  PCopyOutMax=[]  NCopyOutDataTypeStr=Inherit: Inherit via back propagation  NCopyOutMin=[]  NCopyOutMax=[]  IntegratorContinuousStateAttributes=''  IntegratorStateMustResolveToSignalObject=off  IntegratorRTWStateStorageClass=Auto  FilterContinuousStateAttributes=''  FilterStateMustResolveToSignalObject=off  FilterRTWStateStorageClass=Auto  ParallelPVariant=InternalParameters  IdealPVariant=Disabled  IVariant=InternalParameters  DVariant=Disabled  IntegratorVariant=Discrete  SatVariant=Disabled  AWVariant=Passthrough  PCopyVariant=Disabled  TRVariant=Disabled  FdbkBlocksVariant=Forward  IdealPFdbkVariant=Disabled  SatFdbkVariant=Disabled  DerivativeFilterVariant=Disabled  NVariant=Disabled  NCopyVariant=Disabled_SignalSpec  FilterICVariant=Disabled  IntegratorICVariant=InternalICs  ExternalResetVariant=Disabled  TRSumVariant=Passthrough  SumFdbkVariant=Disabled  SumVariant=Sum_PI  TsampFilterVariant=InternalTs  TsampNgainVariant=Passthrough  TsampIntegralVariant=Disabled_SignalSpec  ExternalSaturationOutDataTypeStr=Inherit: Same as second input  DerivativeSourceVariant=Disabled  PreIntVariant=InternalPreInt
  PLL (3ph) : spsPLL3phLib/PLL (3ph)  Fmin=45  Par_Init=[0, 60]  ParK=[180, 3200, 1]  TcD=1e-4  MaxRateChangeFreq=12  FilterCutOffFreq=25  Ts=Ts  AGC=on
  PWM Generator (2-Level) : spsPWMGenerator2LevelLib/PWM Generator (2-Level)  ModulatorType=Three-phase bridge (6 pulses)  ModulatorMode=Unsynchronized  Fc=5e3  Pc=90  nF=27  MinMax="[ -1  1 ]"  SamplingTechnique=Natural  ModulatingSignals=off  m=0.8  Freq=60  Phase=0  Ts=Ts  ShowCarrierOutport=off
  "Power (3ph, Instantaneous)" : spsPower3phInstantaneousLib/Power (3ph, Instantaneous)
  Saturation1 : Saturate  UpperLimit=1.2  LowerLimit=-1.2
  Saturation3 : Saturate  UpperLimit=1.2  LowerLimit=-1.2
  Sum1 : Sum  Inputs=|+-
  Sum2 : Sum  Inputs=|+-
  THD : spsTHDLib/THD  Freq=f  Ts=Ts
  abc to dq0 : spsabctodq0Lib/abc to dq0  Alignment=90 degrees behind phase A axis
  dq0 to abc : spsdq0toabcLib/dq0 to abc  Alignment=90 degrees behind phase A axis
  tag scope: Pinv=global, Qinv=global, THDi=global, d_m=global, i_d=global, i_q=global, m=global, puls_inv=global, q_m=global, wt=global
  wires:
  PID Controller1/1 -> Saturation1/1
  [m] -> PWM Generator (2-Level)/1
  PWM Generator (2-Level)/1 -> [puls_inv]
  Saturation3/1 -> [q_m]
  PID Controller2/1 -> Saturation3/1
  Sum2/1 -> PID Controller2/1
  Demux/1 -> [i_d]
  [Id_ref] -> Sum1/1
  Constant4/1 -> Mux/3
  "Power (3ph, Instantaneous)"/2 -> Gain5/1
  [i_q] -> Sum2/2
  "Power (3ph, Instantaneous)"/1 -> Gain4/1
  [Vabc] -> "Power (3ph, Instantaneous)"/1
  [wt] -> abc to dq0/2
  Saturation1/1 -> [d_m]
  Gain4/1 -> [Pinv]
  Demux/2 -> [i_q]
  [i_d] -> Sum1/2
  Gain5/1 -> [Qinv]
  [Iabc] -> abc to dq0/1
  Sum1/1 -> PID Controller1/1
  Constant3/1 -> Sum2/1
  [Vabc] -> PLL (3ph)/1
  [Iabc] -> "Power (3ph, Instantaneous)"/2
  [d_m] -> Mux/1
  Demux1/1 -> THD/1
  [q_m] -> Mux/2
  PLL (3ph)/2 -> [wt]
  dq0 to abc/1 -> [m]
  abc to dq0/1 -> Demux/1
  [wt] -> dq0 to abc/2
  THD/1 -> Gain2/1
  Gain2/1 -> [THDi]
  [Iabc] -> Demux1/1
  Mux/1 -> dq0 to abc/1

== matlab function newfullgrid/Controller/battery_current_control ==
  data: pv_power input; load_Power input; bat_voltage input; SOC_min input; SOC_max input; Bat_soc input
function fcn(pv_power, load_Power, bat_voltage, SOC_min, SOC_max, Bat_soc)
% Define system parameters
%Ppv      % Power from PV (to be defined based on input from Simulink)
%Pload    % Load demand (to be defined based on input from Simulink)
%Bat_soc  % State of Charge of the battery (input from the battery model)
%SOC_min  % Minimum SOC level allowed
%SOC_max  % Maximum SOC level allowed

% Control Logic
if pv_power > load_Power
    % Case when PV output is greater than Load demand
    if Bat_soc >= SOC_max
        Battery_controling_current = 0 ; % Do not charge the battery for better use of it
        % Export surplus power to the grid if SOC is at max level
        disp('Exporting surplus power to the grid');
    else
        % Charge the battery if SOC is below max level
        disp('Charging batteries');
        % code to charge the battery
        Battery_controling_current = (( pv_power - load_Power) * 1000) / bat_voltage ; 
    end
else
    % Case when PV output is less than Load demand
    if Bat_soc > SOC_min
        % Discharge the battery if SOC is above minimum level
        disp('Discharging batteries');
        % code to discharge the battery
        Battery_controling_current = (( pv_power - load_Power) * 1000) / bat_voltage ; 
    else
        % Import power from the grid to supply the load
        disp('Importing power from the grid');
         Battery_controling_current = 0 ; % Do not discharge the battery for better use of it
       
    end
end

== matlab function newfullgrid/MMPT/MATLAB Function ==
  data: V input; duty output; I input; deltaD_in input
function duty = MPPT_Kontrol( V, I,deltaD_in)

duty_init = 0.05;
duty_min=0;
duty_max=0.75;

persistent Vold Pold duty_old;

if isempty(Vold)
    Vold=0;
    Pold=0;
    duty_old=duty_init;
end
P= V*I;
dV= V - Vold;
dP= P - Pold;
duty = duty_old;
deltaD=deltaD_in;

if dP ~= 0
    if dP < 0
        if dV < 0
            duty = duty_old - deltaD;
        else
            duty = duty_old + deltaD;
        end
    else
        if dV < 0
            duty = duty_old + deltaD;
        else
            duty = duty_old - deltaD;
        end
    end
end

if duty >= duty_max
    duty=duty_max;
elseif duty<duty_min
    duty=duty_min;
end

duty_old=duty;
Vold=V;
Pold=P;

== matlab function newfullgrid/Controller/MATLAB Function ==
  data: pv_power input; pv_power output; load_Power input; bat_voltage input; SOC_min input; SOC_max input; Bat_soc input; load_Power output; bat_voltage output; SOC_min output; SOC_max output; Bat_soc output
function [pv_power, load_Power, bat_voltage, SOC_min, SOC_max, Bat_soc] = downsample_all_inputs(pv_power, load_Power, bat_voltage, SOC_min, SOC_max, Bat_soc)
    % Define the downsample factor
    downsample_factor = 1000; % Adjust this value as necessary

    % Downsample each input
    pv_power = pv_power(1:downsample_factor:end);
    load_Power = load_Power(1:downsample_factor:end);
    bat_voltage = bat_voltage(1:downsample_factor:end);
    SOC_min = SOC_min(1:downsample_factor:end);
    SOC_max = SOC_max(1:downsample_factor:end);
    Bat_soc = Bat_soc(1:downsample_factor:end);
end

== matlab function newfullgrid/Controller/reward  ==
  data: pv_power input; load_power input; soc_min input; soc_max input; bat_soc input; reward output


% 
function reward = rewardFcn(pv_power, load_power, soc_min, soc_max, bat_soc)
    % Inputs:
    %   pv_power   - Power from PV
    %   load_power - Load demand
    %   soc_min    - Minimum SOC level
    %   soc_max    - Maximum SOC level
    %   bat_soc    - Current SOC of the battery
    % Output:
    %   reward     - Scalar normalized reward value

    % Initialize reward
    reward = 0;

    % Maximum absolute reward to normalize scaling
    max_abs_reward = 100;



   if pv_power > load_power
    if bat_soc >= soc_max
        reward = reward + 100; % Higher reward for exporting
    else
        reward = reward + 150; % Higher reward for charging
    end
elseif pv_power < load_power
    if bat_soc > soc_min
        reward = reward + 60; % Moderate reward for discharging
    else
        reward = reward - 150; % Large penalty for grid import
    end
   end


    % Normalize reward to the range [-1, 1]
    reward = reward / max_abs_reward;

    % Ensure the reward is scalar and numeric
    reward = double(reward);
end
% 
% % 
% % 
% % 
% 
% % function reward = rewardFcn(pv_power, load_power, soc_min, soc_max, bat_soc)
% %     % Inputs:
% %     %   pv_power   - Power from PV
% %     %   load_power - Load demand
% %     %   soc_min    - Minimum SOC level
% %     %   soc_max    - Maximum SOC level
% %     %   bat_soc    - Current SOC of the battery
% %     % Output:
% %     %   reward     - Scalar normalized reward value
% % 
% %     % Initialize reward
% %     reward = 0;
% % 
% %     % Maximum absolute reward to normalize scaling
% %     max_abs_reward = 50;
% % 
% %     % Case 1: PV power exceeds load demand
% %     if pv_power > load_power
% %         % SOC at max, export surplus
% %         if bat_soc >= soc_max
% %             reward = reward + 10; % Small reward for exporting power
% %             disp('Reward: Exporting surplus power to the grid.');
% %         else
% %             % SOC below max, encourage charging
% %             reward = reward + 20; % Higher reward for charging battery
% %             disp('Reward: Charging battery.');
% %         end
% %     end
% % 
% %     % Case 2: Load demand exceeds PV power
% %     if pv_power < load_power
% %         % SOC above minimum, encourage discharging
% %         if bat_soc > soc_min
% %             reward = reward + 15; % Reward for discharging battery
% %             disp('Reward: Discharging battery.');
% %         else
% %             % SOC below minimum, penalize grid import
% %             reward = reward - 30; % Penalty for grid import
% %             disp('Penalty: Importing power from the grid.');
% %         end
% %     end
% % 
% %     % Penalize SOC out of bounds
% %     if bat_soc < soc_min
% %         reward = reward - 50; % High penalty for SOC below minimum
% %         disp('Penalty: SOC below minimum.');
% %     elseif bat_soc > soc_max
% %         reward = reward - 50; % High penalty for SOC above maximum
% %         disp('Penalty: SOC above maximum.');
% %     end
% % % 
% % %     % Normalize reward to the range [-1, 1]
% %     reward = reward / max_abs_reward;
% % 
% %     % Ensure the reward is scalar and numeric
% %     reward = double(reward);
% % end

%%%%%%%%%%%%%%%%%

% % 
% function reward = rewardFcn(pv_power, load_power, soc_min, soc_max, bat_soc)
%     % Inputs:
%     %   pv_power   - Power from PV
%     %   load_power - Load demand
%     %   bat_voltage - Battery voltage
%     %   soc_min    - Minimum SOC level
%     %   soc_max    - Maximum SOC level
%     %   bat_soc    - Current SOC of the battery
%     % Output:
%     %   reward     - Scalar reward value
% 
%     % Initialize reward
%     reward = 0;
% 
%     % Case 1: PV power exceeds load demand
%     if pv_power > load_power
%         % SOC at max, export surplus
%         if bat_soc >= soc_max
%             reward = reward + 10; % Small reward for exporting power
%             disp('Reward: Exporting surplus power to the grid.');
%         else
%             % SOC below max, encourage charging
%             reward = reward + 20; % Higher reward for charging battery
%             disp('Reward: Charging battery.');
%         end
%     end
% 
%     % Case 2: Load demand exceeds PV power
%     if pv_power < load_power
%         % SOC above minimum, encourage discharging
%         if bat_soc > soc_min
%             reward = reward + 15; % Reward for discharging battery
%             disp('Reward: Discharging battery.');
%         else
%             % SOC below minimum, penalize grid import
%             reward = reward - 30; % Penalty for grid import
%             disp('Penalty: Importing power from the grid.');
%         end
%     end
% 
%     % Penalize SOC out of bounds
%     if bat_soc < soc_min
%         reward = reward - 50; % High penalty for SOC below minimum
%         disp('Penalty: SOC below minimum.');
%     elseif bat_soc > soc_max
%         reward = reward - 50; % High penalty for SOC above maximum
%         disp('Penalty: SOC above maximum.');
%     end
% end

== matlab function newfullgrid/Controller/isDone ==
  data: Bat_soc input; SOC_min input; SOC_max input; done output
% function isdone = fcnIsDone(SOC_min, SOC_max, Bat_soc)
%     % Check if SOC is out of allowable range
%     if Bat_soc < SOC_min || Bat_soc > SOC_max
%         isdone = true; % End the episode
%     else
%         isdone = false; % Continue the episode
%     end
% end

%%%%%%
% function isdone = fcnIsDone(SOC_min, SOC_max, Bat_soc)
%     % Only end episode if SOC is out of bounds
%     if Bat_soc < SOC_min || Bat_soc > SOC_max
%         isdone = true; % End the episode
%     else
%         isdone = false; % Continue the episode
%     end
% end
%%%%%%%

function done = isdoneFunction(Bat_soc, SOC_min, SOC_max)
    if Bat_soc < SOC_min || Bat_soc > SOC_max
        done = true; % Episode ends when SOC is out of range
    else
        done = false; % Continue episode
    end
end
